simulink model "DCMOTOR"  (R2020a)
settings: Solver=VariableStepAuto  StartTime=0.0  StopTime=10  RelTol=1e-3
values from neighbouring files (symbols this model uses):
  b = 0.1    [MCC.m]
  J = 0.01    [MCC.m]
  K = 0.01    [MCC.m]
  L = 0.5    [MCC.m]
  R = 1    [MCC.m]
settings Model: Creator=Houda Assad

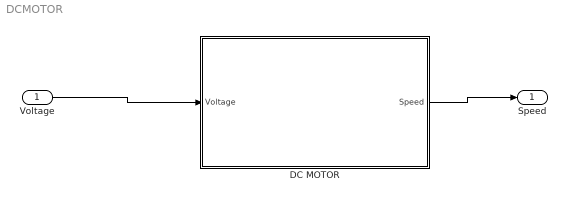
== system DCMOTOR ==
  Voltage : Inport
  DC MOTOR : Subsystem
  Speed : Outport
  wires:
  Voltage/1 -> DC MOTOR/1(Voltage)
  DC MOTOR/1(Speed) -> Speed/1

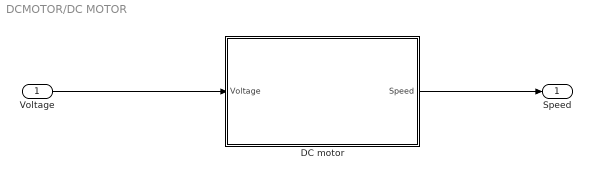
== system DCMOTOR/DC MOTOR ==
  Voltage : Inport
  DC motor : Subsystem
  Speed : Outport
  wires:
  Voltage/1 -> DC motor/1(Voltage)
  DC motor/1(Speed) -> Speed/1

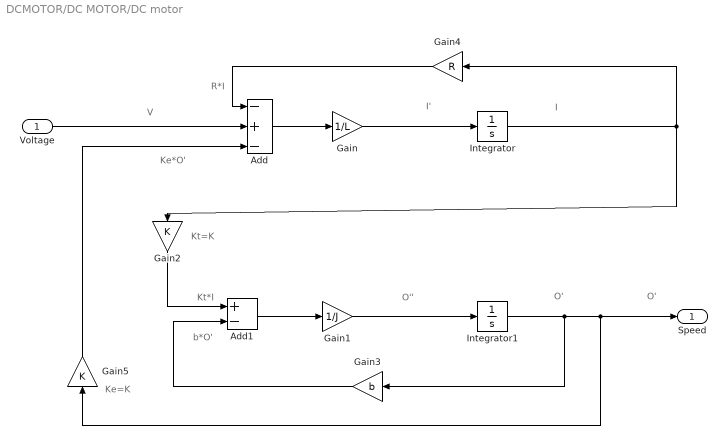
== system DCMOTOR/DC MOTOR/DC motor ==
  note: O'
  note: b*O'
  note: Kt*I
  note: Kt=K
  note: Ke=K
  note: Ke*O'
  note: V
  note: R*I
  note: I'
  note: I
  note: O''
  note: O'
  Voltage : Inport
  Add : Sum  Inputs=-+-
  Add1 : Sum  Inputs=+-
  Gain : Gain  Gain=1/L
  Gain1 : Gain  Gain=1/J
  Gain2 : Gain  Gain=K
  Gain3 : Gain  Gain=b
  Gain4 : Gain  Gain=R
  Gain5 : Gain  Gain=K
  Integrator : Integrator
  Integrator1 : Integrator
  Speed : Outport
  wires:
  Gain3/1 -> Add1/2
  Integrator1/1 -> Speed/1, Gain5/1, Gain3/1
  Gain1/1 -> Integrator1/1
  Add/1 -> Gain/1
  Gain4/1 -> Add/1
  Add1/1 -> Gain1/1
  Gain/1 -> Integrator/1
  Integrator/1 -> Gain4/1, Gain2/1
  Gain2/1 -> Add1/1
  Gain5/1 -> Add/3
  Voltage/1 -> Add/2
